simulink model "APP_MyApplication"  (R2018b)
settings: Solver=VariableStepDiscrete  StartTime=0.0  StopTime=10  RelTol=1e-3
PreLoadFcn:
  | if(exist('MBDS_ModelCallback', 'file')), MBDS_ModelCallback('PreLoad'); end;
PostLoadFcn:
  | if(exist('MBDS_ModelCallback', 'file')), MBDS_ModelCallback('PostLoad'); end;
InitFcn:
  | if(exist('MBDS_ModelCallback', 'file')), MBDS_ModelCallback('Init'); end;
StartFcn:
  | if(exist('MBDS_ModelCallback', 'file')), MBDS_ModelCallback('Start'); end;
StopFcn:
  | if(exist('MBDS_ModelCallback', 'file')), MBDS_ModelCallback('Stop'); end;
undefined symbols (not defined in the file): sigbuilder_block, Ts
libraries: KIBES_Signal x499, simulink x8
(part 4 of 10)

== system APP_MyApplication/Model/APP_MyApplication_/DTC List ==
  note: array
  Constant1 : Constant  InitFcn=|  Value=10  OutDataTypeStr=uint8
      | if(exist('MBDS_BlockCallback', 'file'))
      |    MBDS_BlockCallback('Update', gcb);  
      | end
  Constant7 : Constant  InitFcn=|  OutDataTypeStr=uint8
      | if(exist('MBDS_BlockCallback', 'file'))
      |    MBDS_BlockCallback('Update', gcb);  
      | end
  OR1 : Subsystem  InitFcn=|  mask(OR){MBDS_LibraryBlock=on, BitwiseMode=off, Inputs=2, UseBitMask=off, BitMask='A1', OutDataTypeStr=Inherit: Inherit via back propagation, MBDS_BlockVersion=07.21.05}
      | if(exist('MBDS_BlockCallback', 'file'))
      |    MBDS_BlockCallback('Update', gcb);
      | end
      mask prompts: MBDS_LibraryBlock "MBDS library block"; BitwiseMode "Use 'bitwise' mode"; Inputs "Number of input ports:"; UseBitMask "Use bit mask"; BitMask "Bit mask:"; OutDataTypeStr "Output data type:"; MBDS_BlockVersion "Version:"
      mask help: Logical or bitwise OR operator. For multiple inputs, operators are applied across the inputs. For a single input, operators are applied across the input vector. In bitwise mode a bit mask can be applied onto single input signals.
      mask init: same as APP_MyApplication/Model/APP_MyApplication_/OR
      mask Help: eval(['open([workdir(''library_dir:''),''\Blockset\help\'',get_param(gcb,''MaskType''),''.html''])'])
      mask Callback BitwiseMode:
      | if(exist('MBDS_BlockCallback', 'file'))
      |    MBDS_BlockCallback('BitwiseMode', gcb);
      | end
      mask Callback Inputs:
      | if(exist('MBDS_BlockCallback', 'file'))
      |    MBDS_BlockCallback('Inputs', gcb);
      | end
      mask Callback UseBitMask:
      | if(exist('MBDS_BlockCallback', 'file'))
      |    MBDS_BlockCallback('UseBitMask', gcb);
      | end
      mask Callback BitMask:
      | if(exist('MBDS_BlockCallback', 'file'))
      |    MBDS_BlockCallback('BitMask', gcb);
      | end
      mask TypeOptions OutDataTypeStr: Inherit: Inherit via back propagation | int8 | uint8 | int16 | uint16 | int32 | uint32 | boolean
      mask Callback OutDataTypeStr:
      | % Adopt Value
      | if(exist('MBDS_BlockCallback', 'file'))
      |    MBDS_BlockCallback('OutDataTypeStr', gcb);
      | end
      mask DialogControl ParameterTabVar0 Prompt: Main
      mask DialogControl ParameterTabVar01 Prompt: Signal Attributes
      mask DialogControl ParameterTabVar012 Prompt: Version
      mask Display:
      | % Show icon or block text
      | if(UseBitMask)
      |    if(isnumeric(BitMask))
      |       BitMaskString = ['0x',dec2hex(floor(BitMask))];
      |    elseif(ischar(BitMask))
      |       BitMaskString = ['0x',upper(BitMask)];
      |    else
      |       BitMaskString = '???';
      |    end
      |    disp(sprintf(['OR\n', BitMaskString]))
      | else
      |    disp('OR')
      | end
  in_DtcList.DTCList.DTClistType : KIBES_Signal/KIBES_Signal  MBDS_LibraryBlock=on  DatabaseKey=268  SignalName=DtcList.DTCList.DTClistType  SymbolName=DtcList_DTCList_DTClistType_000268  DataType=uint8  Init=[0 0 0 0 0 0 0 0 0 0]  Slope=1  Bias=0  DataSize=10  fpDataType=uint8  BlockIOType=Inport  DeviceType=0
  in_DtcList.DTCList.f_DTClistECUaddress : KIBES_Signal/KIBES_Signal  MBDS_LibraryBlock=on  DatabaseKey=241  SignalName=DtcList.DTCList.f_DTClistECUaddress  SymbolName=DtcList_DTCList_f_DTClistECUaddress_000241  DataType=uint8  Init=[0 0 0 0 0 0 0 0 0 0]  Slope=1  Bias=0  DataSize=10  fpDataType=uint8  BlockIOType=Inport  DeviceType=0
  in_DtcList.DTCList.f_DTClistFMI : KIBES_Signal/KIBES_Signal  MBDS_LibraryBlock=on  DatabaseKey=245  SignalName=DtcList.DTCList.f_DTClistFMI  SymbolName=DtcList_DTCList_f_DTClistFMI_000245  DataType=uint8  Init=[0 0 0 0 0 0 0 0 0 0]  Slope=1  Bias=0  DataSize=10  fpDataType=uint8  BlockIOType=Inport  DeviceType=0
  in_DtcList.DTCList.f_DTClistFirstEntry : KIBES_Signal/KIBES_Signal  MBDS_LibraryBlock=on  DatabaseKey=244  SignalName=DtcList.DTCList.f_DTClistFirstEntry  SymbolName=DtcList_DTCList_f_DTClistFirstEntry_000244  DataType=boolean  Init=0  Slope=1  Bias=0  DataSize=1  fpDataType=boolean  BlockIOType=Inport  DeviceType=0
  in_DtcList.DTCList.f_DTClistLastEntry : KIBES_Signal/KIBES_Signal  MBDS_LibraryBlock=on  DatabaseKey=246  SignalName=DtcList.DTCList.f_DTClistLastEntry  SymbolName=DtcList_DTCList_f_DTClistLastEntry_000246  DataType=boolean  Init=0  Slope=1  Bias=0  DataSize=1  fpDataType=boolean  BlockIOType=Inport  DeviceType=0
  in_DtcList.DTCList.f_DTClistNumOfEntries : KIBES_Signal/KIBES_Signal  MBDS_LibraryBlock=on  DatabaseKey=248  SignalName=DtcList.DTCList.f_DTClistNumOfEntries  SymbolName=DtcList_DTCList_f_DTClistNumOfEntries_000248  DataType=uint16  Init=0  Slope=1  Bias=0  DataSize=1  fpDataType=uint16  BlockIOType=Inport  DeviceType=0
  in_DtcList.DTCList.f_DTClistOCC : KIBES_Signal/KIBES_Signal  MBDS_LibraryBlock=on  DatabaseKey=249  SignalName=DtcList.DTCList.f_DTClistOCC  SymbolName=DtcList_DTCList_f_DTClistOCC_000249  DataType=uint8  Init=[0 0 0 0 0 0 0 0 0 0]  Slope=1  Bias=0  DataSize=10  fpDataType=uint8  BlockIOType=Inport  DeviceType=0
  in_DtcList.DTCList.f_DTClistPrio : KIBES_Signal/KIBES_Signal  MBDS_LibraryBlock=on  DatabaseKey=251  SignalName=DtcList.DTCList.f_DTClistPrio  SymbolName=DtcList_DTCList_f_DTClistPrio_000251  DataType=uint8  Init=[0 0 0 0 0 0 0 0 0 0]  Slope=1  Bias=0  DataSize=10  fpDataType=uint8  BlockIOType=Inport  DeviceType=0
  in_DtcList.DTCList.f_DTClistSPN : KIBES_Signal/KIBES_Signal  MBDS_LibraryBlock=on  DatabaseKey=252  SignalName=DtcList.DTCList.f_DTClistSPN  SymbolName=DtcList_DTCList_f_DTClistSPN_000252  DataType=uint32  Init=[0 0 0 0 0 0 0 0 0 0]  Slope=1  Bias=0  DataSize=10  fpDataType=uint32  BlockIOType=Inport  DeviceType=0
  in_IN_DIG_02_DriverDoor : KIBES_Signal/KIBES_Signal  MBDS_LibraryBlock=on  DatabaseKey=215  SignalName=IN_DIG_02_DriverDoor  SymbolName=IN_DIG_02_DriverDoor_000215  DataType=boolean  Init=0  Slope=1  Bias=0  DataSize=1  fpDataType=boolean  BlockIOType=Inport  DeviceType=0
  in_STIMD.ListDtcEcuAddrMask : KIBES_Signal/KIBES_Signal  MBDS_LibraryBlock=on  DatabaseKey=254  SignalName=STIMD.ListDtcEcuAddrMask  SymbolName=STIMD_ListDtcEcuAddrMask_000254  DataType=uint8  Init=255  Slope=1  Bias=0  DataSize=1  fpDataType=uint8  BlockIOType=Inport  DeviceType=2
  in_STIMD.ListDtcEnable : KIBES_Signal/KIBES_Signal  MBDS_LibraryBlock=on  DatabaseKey=255  SignalName=STIMD.ListDtcEnable  SymbolName=STIMD_ListDtcEnable_000255  DataType=boolean  Init=0  Slope=1  Bias=0  DataSize=1  fpDataType=boolean  BlockIOType=Inport  DeviceType=2
  in_STIMD.ListDtcNextEntry : KIBES_Signal/KIBES_Signal  MBDS_LibraryBlock=on  DatabaseKey=256  SignalName=STIMD.ListDtcNextEntry  SymbolName=STIMD_ListDtcNextEntry_000256  DataType=boolean  Init=0  Slope=1  Bias=0  DataSize=1  fpDataType=boolean  BlockIOType=Inport  DeviceType=2
  in_STIMD.ListDtcPrevEntry : KIBES_Signal/KIBES_Signal  MBDS_LibraryBlock=on  DatabaseKey=257  SignalName=STIMD.ListDtcPrevEntry  SymbolName=STIMD_ListDtcPrevEntry_000257  DataType=boolean  Init=0  Slope=1  Bias=0  DataSize=1  fpDataType=boolean  BlockIOType=Inport  DeviceType=2
  in_STIMD.ListDtcSelectCanChannel : KIBES_Signal/KIBES_Signal  MBDS_LibraryBlock=on  DatabaseKey=450  SignalName=STIMD.ListDtcSelectCanChannel  SymbolName=STIMD_ListDtcSelectCanChannel_000450  DataType=uint8  Init=10  Slope=1  Bias=0  DataSize=1  fpDataType=uint8  BlockIOType=Inport  DeviceType=2
  in_STIMD.ListDtcStatusMask : KIBES_Signal/KIBES_Signal  MBDS_LibraryBlock=on  DatabaseKey=258  SignalName=STIMD.ListDtcStatusMask  SymbolName=STIMD_ListDtcStatusMask_000258  DataType=uint8  Init=1  Slope=1  Bias=0  DataSize=1  fpDataType=uint8  BlockIOType=Inport  DeviceType=2
  out_DtcList.DTCList.SelectCANChannel : KIBES_Signal/KIBES_Signal  MBDS_LibraryBlock=on  DatabaseKey=269  SignalName=DtcList.DTCList.SelectCANChannel  SymbolName=DtcList_DTCList_SelectCANChannel_000269  DataType=uint8  Init=0  Slope=1  Bias=0  DataSize=1  fpDataType=uint8  BlockIOType=Outport  DeviceType=0
  out_DtcList.DTCList.f_DTClistECUaddrMask : KIBES_Signal/KIBES_Signal  MBDS_LibraryBlock=on  DatabaseKey=242  SignalName=DtcList.DTCList.f_DTClistECUaddrMask  SymbolName=DtcList_DTCList_f_DTClistECUaddrMask_000242  DataType=uint8  Init=0  Slope=1  Bias=0  DataSize=1  fpDataType=uint8  BlockIOType=Outport  DeviceType=0
  out_DtcList.DTCList.f_DTClistEna : KIBES_Signal/KIBES_Signal  MBDS_LibraryBlock=on  DatabaseKey=243  SignalName=DtcList.DTCList.f_DTClistEna  SymbolName=DtcList_DTCList_f_DTClistEna_000243  DataType=boolean  Init=0  Slope=1  Bias=0  DataSize=1  fpDataType=boolean  BlockIOType=Outport  DeviceType=0
  out_DtcList.DTCList.f_DTClistNextEntry : KIBES_Signal/KIBES_Signal  MBDS_LibraryBlock=on  DatabaseKey=247  SignalName=DtcList.DTCList.f_DTClistNextEntry  SymbolName=DtcList_DTCList_f_DTClistNextEntry_000247  DataType=boolean  Init=0  Slope=1  Bias=0  DataSize=1  fpDataType=boolean  BlockIOType=Outport  DeviceType=0
  out_DtcList.DTCList.f_DTClistPrevEntry : KIBES_Signal/KIBES_Signal  MBDS_LibraryBlock=on  DatabaseKey=250  SignalName=DtcList.DTCList.f_DTClistPrevEntry  SymbolName=DtcList_DTCList_f_DTClistPrevEntry_000250  DataType=boolean  Init=0  Slope=1  Bias=0  DataSize=1  fpDataType=boolean  BlockIOType=Outport  DeviceType=0
  out_DtcList.DTCList.f_DTClistStatusMask : KIBES_Signal/KIBES_Signal  MBDS_LibraryBlock=on  DatabaseKey=253  SignalName=DtcList.DTCList.f_DTClistStatusMask  SymbolName=DtcList_DTCList_f_DTClistStatusMask_000253  DataType=uint8  Init=0  Slope=1  Bias=0  DataSize=1  fpDataType=uint8  BlockIOType=Outport  DeviceType=0
  wires:
  in_STIMD.ListDtcEcuAddrMask/1 -> out_DtcList.DTCList.f_DTClistECUaddrMask/1
  in_STIMD.ListDtcNextEntry/1 -> out_DtcList.DTCList.f_DTClistNextEntry/1
  in_STIMD.ListDtcPrevEntry/1 -> out_DtcList.DTCList.f_DTClistPrevEntry/1
  OR1/1(y) -> out_DtcList.DTCList.f_DTClistEna/1
  in_STIMD.ListDtcEnable/1 -> OR1/1(u1)
  in_IN_DIG_02_DriverDoor/1 -> OR1/2(u2)
  in_STIMD.ListDtcStatusMask/1 -> out_DtcList.DTCList.f_DTClistStatusMask/1
  in_STIMD.ListDtcSelectCanChannel/1 -> out_DtcList.DTCList.SelectCANChannel/1

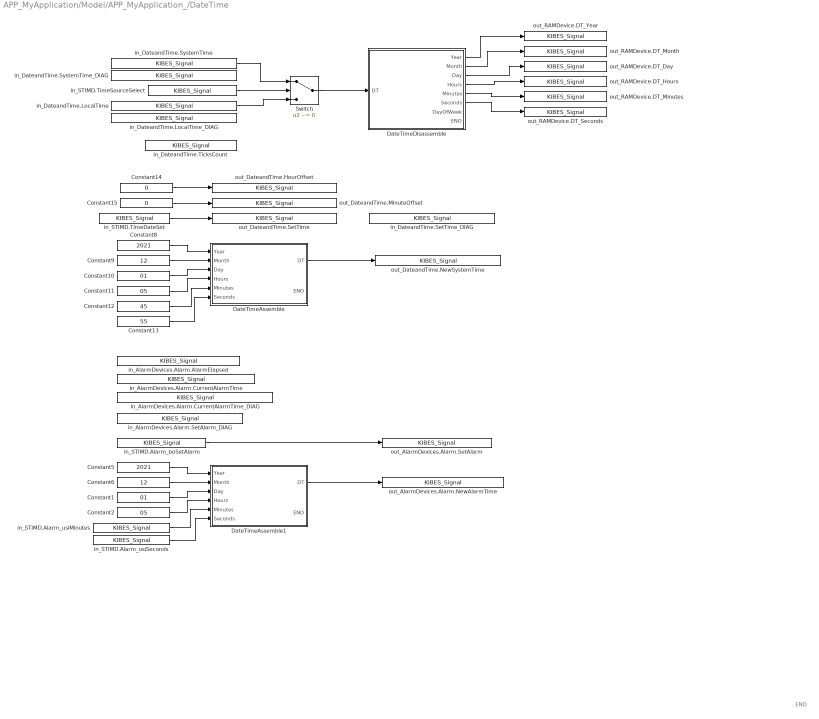
== system APP_MyApplication/Model/APP_MyApplication_/DateTime ==
  note: END
  Constant1 : Constant  InitFcn=|  Value=01  OutDataTypeStr=uint8
      | if(exist('MBDS_BlockCallback', 'file'))
      |    MBDS_BlockCallback('Update', gcb);  
      | end
  Constant10 : Constant  InitFcn=|  Value=01  OutDataTypeStr=uint8
      | if(exist('MBDS_BlockCallback', 'file'))
      |    MBDS_BlockCallback('Update', gcb);  
      | end
  Constant11 : Constant  InitFcn=|  Value=05  OutDataTypeStr=uint8
      | if(exist('MBDS_BlockCallback', 'file'))
      |    MBDS_BlockCallback('Update', gcb);  
      | end
  Constant12 : Constant  InitFcn=|  Value=45  OutDataTypeStr=uint8
      | if(exist('MBDS_BlockCallback', 'file'))
      |    MBDS_BlockCallback('Update', gcb);  
      | end
  Constant13 : Constant  InitFcn=|  Value=55  OutDataTypeStr=uint8
      | if(exist('MBDS_BlockCallback', 'file'))
      |    MBDS_BlockCallback('Update', gcb);  
      | end
  Constant14 : Constant  InitFcn=|  Value=0  OutDataTypeStr=int8
      | if(exist('MBDS_BlockCallback', 'file'))
      |    MBDS_BlockCallback('Update', gcb);  
      | end
  Constant15 : Constant  InitFcn=|  Value=0  OutDataTypeStr=int8
      | if(exist('MBDS_BlockCallback', 'file'))
      |    MBDS_BlockCallback('Update', gcb);  
      | end
  Constant2 : Constant  InitFcn=|  Value=05  OutDataTypeStr=uint8
      | if(exist('MBDS_BlockCallback', 'file'))
      |    MBDS_BlockCallback('Update', gcb);  
      | end
  Constant5 : Constant  InitFcn=|  Value=2021  OutDataTypeStr=uint16
      | if(exist('MBDS_BlockCallback', 'file'))
      |    MBDS_BlockCallback('Update', gcb);  
      | end
  Constant6 : Constant  InitFcn=|  Value=12  OutDataTypeStr=uint8
      | if(exist('MBDS_BlockCallback', 'file'))
      |    MBDS_BlockCallback('Update', gcb);  
      | end
  Constant8 : Constant  InitFcn=|  Value=2021  OutDataTypeStr=uint16
      | if(exist('MBDS_BlockCallback', 'file'))
      |    MBDS_BlockCallback('Update', gcb);  
      | end
  Constant9 : Constant  InitFcn=|  Value=12  OutDataTypeStr=uint8
      | if(exist('MBDS_BlockCallback', 'file'))
      |    MBDS_BlockCallback('Update', gcb);  
      | end
  DateTimeAssemble : Subsystem  mask(DateTimeAssemble){MBDS_LibraryBlock=on, ENO_Enabled=on, MBDS_BlockVersion=07.21.06}
      mask prompts: MBDS_LibraryBlock "MBDS library block"; ENO_Enabled "Show ENO port"; MBDS_BlockVersion "Block version:"
      mask help: Assembles a date_time signal from individual date and time components. The input values are restricted to their ranges (refer to the block help). If an input is out of range the ENO output is set to false.
      mask init: same as APP_MyApplication/Model/APP_MyApplication_/OR
      mask Help: eval(['open([workdir(''Library_Dir:''),''\Blockset\Help\'',get_param(gcb,''MaskType''),''.html''])']);
      mask DialogControl Container4 Prompt: Main
      mask DialogControl Container5 Prompt: Version
      mask Display:
      | % Show block text
      | disp(sprintf('DateTime\nAssemble'));
      | 
      | % Display port labels
      | port_label('input', 1, 'Year');
      | port_label('input', 2, 'Month');
      | port_label('input', 3, 'Day');
      | port_label('input', 4, 'Hours');
      | port_label('input', 5, 'Minutes');
      | port_label('input', 6, 'Seconds');
      | port_label('output', 1, 'DT');
      | port_label('output', 2, 'ENO');
  DateTimeAssemble1 : Subsystem  mask(DateTimeAssemble){MBDS_LibraryBlock=on, ENO_Enabled=on, MBDS_BlockVersion=07.21.06}
      mask prompts: MBDS_LibraryBlock "MBDS library block"; ENO_Enabled "Show ENO port"; MBDS_BlockVersion "Block version:"
      mask help: Assembles a date_time signal from individual date and time components. The input values are restricted to their ranges (refer to the block help). If an input is out of range the ENO output is set to false.
      mask init: same as APP_MyApplication/Model/APP_MyApplication_/OR
      mask Help: eval(['open([workdir(''Library_Dir:''),''\Blockset\Help\'',get_param(gcb,''MaskType''),''.html''])']);
      mask DialogControl Container4 Prompt: Main
      mask DialogControl Container5 Prompt: Version
      mask Display:
      | % Show block text
      | disp(sprintf('DateTime\nAssemble'));
      | 
      | % Display port labels
      | port_label('input', 1, 'Year');
      | port_label('input', 2, 'Month');
      | port_label('input', 3, 'Day');
      | port_label('input', 4, 'Hours');
      | port_label('input', 5, 'Minutes');
      | port_label('input', 6, 'Seconds');
      | port_label('output', 1, 'DT');
      | port_label('output', 2, 'ENO');
  DateTimeDisassemble : Subsystem  mask(DateTimeDisassemble){MBDS_LibraryBlock=on, ENO_Enabled=on, MBDS_BlockVersion=07.21.06}
      mask prompts: MBDS_LibraryBlock "MBDS library block"; ENO_Enabled "Show ENO port"; MBDS_BlockVersion "Block version:"
      mask help: Disassembles a date_time signal into its date time components, i.e. year, month, day, hour, minute, second. Additionally the day of week number is output. If the input signal is invalid the ENO output is false.
      mask init: same as APP_MyApplication/Model/APP_MyApplication_/OR
      mask Help: eval(['open([workdir(''Library_Dir:''),''\Blockset\Help\'',get_param(gcb,''MaskType''),''.html''])']);
      mask DialogControl Container8 Prompt: Main
      mask DialogControl Container11 Prompt: Version
      mask Display:
      | % Show block text
      | disp(sprintf('DateTime\nDisassemble'));
      | 
      | % Display port labels
      | port_label('input', 1, 'DT');
      | port_label('output', 1, 'Year');
      | port_label('output', 2, 'Month');
      | port_label('output', 3, 'Day');
      | port_label('output', 4, 'Hours');
      | port_label('output', 5, 'Minutes');
      | port_label('output', 6, 'Seconds');
      | port_label('output', 7, 'DayOfWeek');
      | port_label('output', 8, 'ENO');
  Switch : Switch  InitFcn=|  Criteria=u2 ~= 0  OutDataTypeStr=Inherit: Inherit via back propagation  mask(Switch){MBDS_LibraryBlock=on, OutDataTypeStr_=Inherit: Inherit via back propagation, SaturateOnIntegerOverflow_=off, InputSameDT_=off, MBDS_BlockVersion=07.21.05}
      | if(exist('MBDS_BlockCallback', 'file'))
      |    MBDS_BlockCallback('Update', gcb);  
      | end
      mask prompts: MBDS_LibraryBlock "MBDS library block"; OutDataTypeStr_ "Output data type:"; SaturateOnIntegerOverflow_ "Saturate on integer overflow"; InputSameDT_ "Require all inputs to have the same data type"; MBDS_BlockVersion "Block version:"
      mask help: Pass through input 1 when input 2 is not equal to zero; otherwise pass through input 3. The inputs are numbered top to bottom (or left to right). The first and third input ports are data ports, and the second input port is the control port.
      mask init: same as APP_MyApplication/Model/APP_MyApplication_/OR
      mask Help: eval(['open([workdir(''library_dir:''),''\Blockset\help\'',get_param(gcb,''MaskType''),''.html''])'])
      mask TypeOptions OutDataTypeStr_: Inherit: Inherit via back propagation | single | int8 | uint8 | int16 | uint16 | int32 | uint32
      mask DialogControl ParameterTabVar0 Prompt: Signal Attributes
      mask DialogControl ParameterTabVar01 Prompt: Version
  in_AlarmDevices.Alarm.AlarmElapsed : KIBES_Signal/KIBES_Signal  MBDS_LibraryBlock=on  DatabaseKey=621  SignalName=AlarmDevices.Alarm.AlarmElapsed  SymbolName=AlarmDevices_Alarm_AlarmElapsed_000621  DataType=boolean  Init=0  Slope=1  Bias=0  DataSize=1  fpDataType=boolean  BlockIOType=Inport  DeviceType=0
  in_AlarmDevices.Alarm.CurrentAlarmTime : KIBES_Signal/KIBES_Signal  MBDS_LibraryBlock=on  DatabaseKey=623  SignalName=AlarmDevices.Alarm.CurrentAlarmTime  SymbolName=AlarmDevices_Alarm_CurrentAlarmTime_000623  DataType=uint32  Init=0  Slope=1  Bias=0  DataSize=1  fpDataType=uint32  BlockIOType=Inport  DeviceType=0
  in_AlarmDevices.Alarm.CurrentAlarmTime_DIAG : KIBES_Signal/KIBES_Signal  MBDS_LibraryBlock=on  DatabaseKey=624  SignalName=AlarmDevices.Alarm.CurrentAlarmTime_DIAG  SymbolName=AlarmDevices_Alarm_CurrentAlarmTime_DIAG_000624  DataType=uint16  Init=1  Slope=1  Bias=0  DataSize=1  fpDataType=uint16  BlockIOType=Inport  DeviceType=0
  in_AlarmDevices.Alarm.SetAlarm_DIAG : KIBES_Signal/KIBES_Signal  MBDS_LibraryBlock=on  DatabaseKey=634  SignalName=AlarmDevices.Alarm.SetAlarm_DIAG  SymbolName=AlarmDevices_Alarm_SetAlarm_DIAG_000634  DataType=uint16  Init=1  Slope=1  Bias=0  DataSize=1  fpDataType=uint16  BlockIOType=Inport  DeviceType=0
  in_DateandTime.LocalTime : KIBES_Signal/KIBES_Signal  MBDS_LibraryBlock=on  DatabaseKey=415  SignalName=DateandTime.LocalTime  SymbolName=DateandTime_LocalTime_000415  DataType=uint32  Init=0  Slope=1  Bias=0  DataSize=1  fpDataType=uint32  BlockIOType=Inport  DeviceType=0
  in_DateandTime.LocalTime_DIAG : KIBES_Signal/KIBES_Signal  MBDS_LibraryBlock=on  DatabaseKey=418  SignalName=DateandTime.LocalTime_DIAG  SymbolName=DateandTime_LocalTime_DIAG_000418  DataType=uint16  Init=1  Slope=1  Bias=0  DataSize=1  fpDataType=uint16  BlockIOType=Inport  DeviceType=0
  in_DateandTime.SetTime_DIAG : KIBES_Signal/KIBES_Signal  MBDS_LibraryBlock=on  DatabaseKey=410  SignalName=DateandTime.SetTime_DIAG  SymbolName=DateandTime_SetTime_DIAG_000410  DataType=uint16  Init=1  Slope=1  Bias=0  DataSize=1  fpDataType=uint16  BlockIOType=Inport  DeviceType=0
  in_DateandTime.SystemTime : KIBES_Signal/KIBES_Signal  MBDS_LibraryBlock=on  DatabaseKey=412  SignalName=DateandTime.SystemTime  SymbolName=DateandTime_SystemTime_000412  DataType=uint32  Init=0  Slope=1  Bias=0  DataSize=1  fpDataType=uint32  BlockIOType=Inport  DeviceType=0
  in_DateandTime.SystemTime_DIAG : KIBES_Signal/KIBES_Signal  MBDS_LibraryBlock=on  DatabaseKey=413  SignalName=DateandTime.SystemTime_DIAG  SymbolName=DateandTime_SystemTime_DIAG_000413  DataType=uint16  Init=1  Slope=1  Bias=0  DataSize=1  fpDataType=uint16  BlockIOType=Inport  DeviceType=0
  in_DateandTime.TicksCount : KIBES_Signal/KIBES_Signal  MBDS_LibraryBlock=on  DatabaseKey=414  SignalName=DateandTime.TicksCount  SymbolName=DateandTime_TicksCount_000414  DataType=uint32  Init=0  Slope=1  Bias=0  DataSize=1  fpDataType=uint32  BlockIOType=Inport  DeviceType=0
  in_STIMD.Alarm_boSetAlarm : KIBES_Signal/KIBES_Signal  MBDS_LibraryBlock=on  DatabaseKey=627  SignalName=STIMD.Alarm_boSetAlarm  SymbolName=STIMD_Alarm_boSetAlarm_000627  DataType=boolean  Init=0  Slope=1  Bias=0  DataSize=1  fpDataType=boolean  BlockIOType=Inport  DeviceType=2
  in_STIMD.Alarm_usiMinutes : KIBES_Signal/KIBES_Signal  MBDS_LibraryBlock=on  DatabaseKey=628  SignalName=STIMD.Alarm_usiMinutes  SymbolName=STIMD_Alarm_usiMinutes_000628  DataType=uint8  Init=0  Slope=1  Bias=0  DataSize=1  fpDataType=uint8  BlockIOType=Inport  DeviceType=2
  in_STIMD.Alarm_usiSeconds : KIBES_Signal/KIBES_Signal  MBDS_LibraryBlock=on  DatabaseKey=630  SignalName=STIMD.Alarm_usiSeconds  SymbolName=STIMD_Alarm_usiSeconds_000630  DataType=uint8  Init=0  Slope=1  Bias=0  DataSize=1  fpDataType=uint8  BlockIOType=Inport  DeviceType=2
  in_STIMD.TimeDateSet : KIBES_Signal/KIBES_Signal  MBDS_LibraryBlock=on  DatabaseKey=420  SignalName=STIMD.TimeDateSet  SymbolName=STIMD_TimeDateSet_000420  DataType=boolean  Init=0  Slope=1  Bias=0  DataSize=1  fpDataType=boolean  BlockIOType=Inport  DeviceType=2
  in_STIMD.TimeSourceSelect : KIBES_Signal/KIBES_Signal  MBDS_LibraryBlock=on  DatabaseKey=620  SignalName=STIMD.TimeSourceSelect  SymbolName=STIMD_TimeSourceSelect_000620  DataType=boolean  Init=0  Slope=1  Bias=0  DataSize=1  fpDataType=boolean  BlockIOType=Inport  DeviceType=2
  out_AlarmDevices.Alarm.NewAlarmTime : KIBES_Signal/KIBES_Signal  MBDS_LibraryBlock=on  DatabaseKey=625  SignalName=AlarmDevices.Alarm.NewAlarmTime  SymbolName=AlarmDevices_Alarm_NewAlarmTime_000625  DataType=uint32  Init=0  Slope=1  Bias=0  DataSize=1  fpDataType=uint32  BlockIOType=Outport  DeviceType=0
  out_AlarmDevices.Alarm.SetAlarm : KIBES_Signal/KIBES_Signal  MBDS_LibraryBlock=on  DatabaseKey=626  SignalName=AlarmDevices.Alarm.SetAlarm  SymbolName=AlarmDevices_Alarm_SetAlarm_000626  DataType=boolean  Init=0  Slope=1  Bias=0  DataSize=1  fpDataType=boolean  BlockIOType=Outport  DeviceType=0
  out_DateandTime.HourOffset : KIBES_Signal/KIBES_Signal  MBDS_LibraryBlock=on  DatabaseKey=416  SignalName=DateandTime.HourOffset  SymbolName=DateandTime_HourOffset_000416  DataType=int8  Init=0  Slope=1  Bias=0  DataSize=1  fpDataType=int8  BlockIOType=Outport  DeviceType=0
  out_DateandTime.MinuteOffset : KIBES_Signal/KIBES_Signal  MBDS_LibraryBlock=on  DatabaseKey=419  SignalName=DateandTime.MinuteOffset  SymbolName=DateandTime_MinuteOffset_000419  DataType=int8  Init=0  Slope=1  Bias=0  DataSize=1  fpDataType=int8  BlockIOType=Outport  DeviceType=0
  out_DateandTime.NewSystemTime : KIBES_Signal/KIBES_Signal  MBDS_LibraryBlock=on  DatabaseKey=417  SignalName=DateandTime.NewSystemTime  SymbolName=DateandTime_NewSystemTime_000417  DataType=uint32  Init=0  Slope=1  Bias=0  DataSize=1  fpDataType=uint32  BlockIOType=Outport  DeviceType=0
  out_DateandTime.SetTime : KIBES_Signal/KIBES_Signal  MBDS_LibraryBlock=on  DatabaseKey=411  SignalName=DateandTime.SetTime  SymbolName=DateandTime_SetTime_000411  DataType=boolean  Init=0  Slope=1  Bias=0  DataSize=1  fpDataType=boolean  BlockIOType=Outport  DeviceType=0
  out_RAMDevice.DT_Day : KIBES_Signal/KIBES_Signal  MBDS_LibraryBlock=on  DatabaseKey=424  SignalName=RAMDevice.DT_Day  SymbolName=RAMDevice_DT_Day_000424  DataType=uint8  Init=0  Slope=1  Bias=0  DataSize=1  fpDataType=uint8  BlockIOType=Outport  DeviceType=0
  out_RAMDevice.DT_Hours : KIBES_Signal/KIBES_Signal  MBDS_LibraryBlock=on  DatabaseKey=423  SignalName=RAMDevice.DT_Hours  SymbolName=RAMDevice_DT_Hours_000423  DataType=uint8  Init=0  Slope=1  Bias=0  DataSize=1  fpDataType=uint8  BlockIOType=Outport  DeviceType=0
  out_RAMDevice.DT_Minutes : KIBES_Signal/KIBES_Signal  MBDS_LibraryBlock=on  DatabaseKey=425  SignalName=RAMDevice.DT_Minutes  SymbolName=RAMDevice_DT_Minutes_000425  DataType=uint8  Init=0  Slope=1  Bias=0  DataSize=1  fpDataType=uint8  BlockIOType=Outport  DeviceType=0
  out_RAMDevice.DT_Month : KIBES_Signal/KIBES_Signal  MBDS_LibraryBlock=on  DatabaseKey=422  SignalName=RAMDevice.DT_Month  SymbolName=RAMDevice_DT_Month_000422  DataType=uint8  Init=0  Slope=1  Bias=0  DataSize=1  fpDataType=uint8  BlockIOType=Outport  DeviceType=0
  out_RAMDevice.DT_Seconds : KIBES_Signal/KIBES_Signal  MBDS_LibraryBlock=on  DatabaseKey=426  SignalName=RAMDevice.DT_Seconds  SymbolName=RAMDevice_DT_Seconds_000426  DataType=uint8  Init=0  Slope=1  Bias=0  DataSize=1  fpDataType=uint8  BlockIOType=Outport  DeviceType=0
  out_RAMDevice.DT_Year : KIBES_Signal/KIBES_Signal  MBDS_LibraryBlock=on  DatabaseKey=421  SignalName=RAMDevice.DT_Year  SymbolName=RAMDevice_DT_Year_000421  DataType=uint16  Init=0  Slope=1  Bias=0  DataSize=1  fpDataType=uint16  BlockIOType=Outport  DeviceType=0
  wires:
  DateTimeAssemble/1(DT) -> out_DateandTime.NewSystemTime/1
  Constant8/1 -> DateTimeAssemble/1(Year)
  Constant9/1 -> DateTimeAssemble/2(Month)
  Constant10/1 -> DateTimeAssemble/3(Day)
  Constant11/1 -> DateTimeAssemble/4(Hours)
  Constant12/1 -> DateTimeAssemble/5(Minutes)
  Constant13/1 -> DateTimeAssemble/6(Seconds)
  Constant14/1 -> out_DateandTime.HourOffset/1
  Constant15/1 -> out_DateandTime.MinuteOffset/1
  in_STIMD.TimeDateSet/1 -> out_DateandTime.SetTime/1
  DateTimeDisassemble/2(Month) -> out_RAMDevice.DT_Month/1
  DateTimeDisassemble/1(Year) -> out_RAMDevice.DT_Year/1
  DateTimeDisassemble/5(Minutes) -> out_RAMDevice.DT_Minutes/1
  DateTimeDisassemble/4(Hours) -> out_RAMDevice.DT_Hours/1
  DateTimeDisassemble/3(Day) -> out_RAMDevice.DT_Day/1
  DateTimeDisassemble/6(Seconds) -> out_RAMDevice.DT_Seconds/1
  in_DateandTime.SystemTime/1 -> Switch/1
  in_DateandTime.LocalTime/1 -> Switch/3
  Switch/1 -> DateTimeDisassemble/1(DT)
  in_STIMD.TimeSourceSelect/1 -> Switch/2
  Constant2/1 -> DateTimeAssemble1/4(Hours)
  Constant1/1 -> DateTimeAssemble1/3(Day)
  Constant6/1 -> DateTimeAssemble1/2(Month)
  Constant5/1 -> DateTimeAssemble1/1(Year)
  DateTimeAssemble1/1(DT) -> out_AlarmDevices.Alarm.NewAlarmTime/1
  in_STIMD.Alarm_boSetAlarm/1 -> out_AlarmDevices.Alarm.SetAlarm/1
  in_STIMD.Alarm_usiMinutes/1 -> DateTimeAssemble1/5(Minutes)
  in_STIMD.Alarm_usiSeconds/1 -> DateTimeAssemble1/6(Seconds)

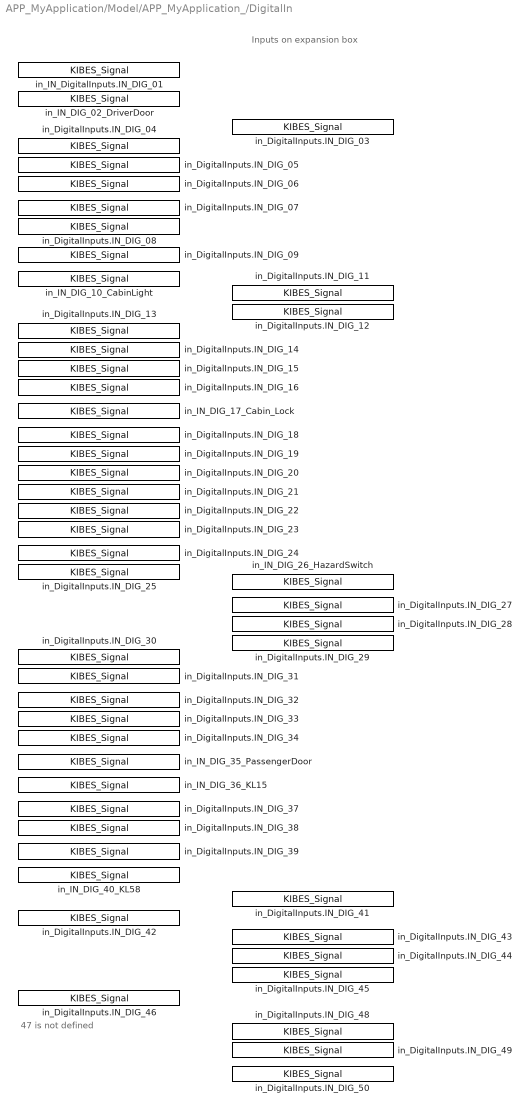
== system APP_MyApplication/Model/APP_MyApplication_/DigitalIn ==
  note: 47 is not defined
  note: Inputs on expansion box
  in_DigitalInputs.IN_DIG_03 : KIBES_Signal/KIBES_Signal  MBDS_LibraryBlock=on  DatabaseKey=456  SignalName=DigitalInputs.IN_DIG_03  SymbolName=DigitalInputs_IN_DIG_03_000456  DataType=boolean  Init=0  Slope=1  Bias=0  DataSize=1  fpDataType=boolean  BlockIOType=Inport  DeviceType=0
  in_DigitalInputs.IN_DIG_04 : KIBES_Signal/KIBES_Signal  MBDS_LibraryBlock=on  DatabaseKey=461  SignalName=DigitalInputs.IN_DIG_04  SymbolName=DigitalInputs_IN_DIG_04_000461  DataType=boolean  Init=0  Slope=1  Bias=0  DataSize=1  fpDataType=boolean  BlockIOType=Inport  DeviceType=0
  in_DigitalInputs.IN_DIG_05 : KIBES_Signal/KIBES_Signal  MBDS_LibraryBlock=on  DatabaseKey=462  SignalName=DigitalInputs.IN_DIG_05  SymbolName=DigitalInputs_IN_DIG_05_000462  DataType=boolean  Init=0  Slope=1  Bias=0  DataSize=1  fpDataType=boolean  BlockIOType=Inport  DeviceType=0
  in_DigitalInputs.IN_DIG_06 : KIBES_Signal/KIBES_Signal  MBDS_LibraryBlock=on  DatabaseKey=463  SignalName=DigitalInputs.IN_DIG_06  SymbolName=DigitalInputs_IN_DIG_06_000463  DataType=boolean  Init=0  Slope=1  Bias=0  DataSize=1  fpDataType=boolean  BlockIOType=Inport  DeviceType=0
  in_DigitalInputs.IN_DIG_07 : KIBES_Signal/KIBES_Signal  MBDS_LibraryBlock=on  DatabaseKey=464  SignalName=DigitalInputs.IN_DIG_07  SymbolName=DigitalInputs_IN_DIG_07_000464  DataType=boolean  Init=0  Slope=1  Bias=0  DataSize=1  fpDataType=boolean  BlockIOType=Inport  DeviceType=0
  in_DigitalInputs.IN_DIG_08 : KIBES_Signal/KIBES_Signal  MBDS_LibraryBlock=on  DatabaseKey=465  SignalName=DigitalInputs.IN_DIG_08  SymbolName=DigitalInputs_IN_DIG_08_000465  DataType=boolean  Init=0  Slope=1  Bias=0  DataSize=1  fpDataType=boolean  BlockIOType=Inport  DeviceType=0
  in_DigitalInputs.IN_DIG_09 : KIBES_Signal/KIBES_Signal  MBDS_LibraryBlock=on  DatabaseKey=457  SignalName=DigitalInputs.IN_DIG_09  SymbolName=DigitalInputs_IN_DIG_09_000457  DataType=boolean  Init=0  Slope=1  Bias=0  DataSize=1  fpDataType=boolean  BlockIOType=Inport  DeviceType=0
  in_DigitalInputs.IN_DIG_11 : KIBES_Signal/KIBES_Signal  MBDS_LibraryBlock=on  DatabaseKey=466  SignalName=DigitalInputs.IN_DIG_11  SymbolName=DigitalInputs_IN_DIG_11_000466  DataType=boolean  Init=0  Slope=1  Bias=0  DataSize=1  fpDataType=boolean  BlockIOType=Inport  DeviceType=0
  in_DigitalInputs.IN_DIG_12 : KIBES_Signal/KIBES_Signal  MBDS_LibraryBlock=on  DatabaseKey=467  SignalName=DigitalInputs.IN_DIG_12  SymbolName=DigitalInputs_IN_DIG_12_000467  DataType=boolean  Init=0  Slope=1  Bias=0  DataSize=1  fpDataType=boolean  BlockIOType=Inport  DeviceType=0
  in_DigitalInputs.IN_DIG_13 : KIBES_Signal/KIBES_Signal  MBDS_LibraryBlock=on  DatabaseKey=468  SignalName=DigitalInputs.IN_DIG_13  SymbolName=DigitalInputs_IN_DIG_13_000468  DataType=boolean  Init=0  Slope=1  Bias=0  DataSize=1  fpDataType=boolean  BlockIOType=Inport  DeviceType=0
  in_DigitalInputs.IN_DIG_14 : KIBES_Signal/KIBES_Signal  MBDS_LibraryBlock=on  DatabaseKey=469  SignalName=DigitalInputs.IN_DIG_14  SymbolName=DigitalInputs_IN_DIG_14_000469  DataType=boolean  Init=0  Slope=1  Bias=0  DataSize=1  fpDataType=boolean  BlockIOType=Inport  DeviceType=0
  in_DigitalInputs.IN_DIG_15 : KIBES_Signal/KIBES_Signal  MBDS_LibraryBlock=on  DatabaseKey=470  SignalName=DigitalInputs.IN_DIG_15  SymbolName=DigitalInputs_IN_DIG_15_000470  DataType=boolean  Init=0  Slope=1  Bias=0  DataSize=1  fpDataType=boolean  BlockIOType=Inport  DeviceType=0
  in_DigitalInputs.IN_DIG_16 : KIBES_Signal/KIBES_Signal  MBDS_LibraryBlock=on  DatabaseKey=471  SignalName=DigitalInputs.IN_DIG_16  SymbolName=DigitalInputs_IN_DIG_16_000471  DataType=boolean  Init=0  Slope=1  Bias=0  DataSize=1  fpDataType=boolean  BlockIOType=Inport  DeviceType=0
  in_DigitalInputs.IN_DIG_18 : KIBES_Signal/KIBES_Signal  MBDS_LibraryBlock=on  DatabaseKey=472  SignalName=DigitalInputs.IN_DIG_18  SymbolName=DigitalInputs_IN_DIG_18_000472  DataType=boolean  Init=0  Slope=1  Bias=0  DataSize=1  fpDataType=boolean  BlockIOType=Inport  DeviceType=0
  in_DigitalInputs.IN_DIG_19 : KIBES_Signal/KIBES_Signal  MBDS_LibraryBlock=on  DatabaseKey=473  SignalName=DigitalInputs.IN_DIG_19  SymbolName=DigitalInputs_IN_DIG_19_000473  DataType=boolean  Init=0  Slope=1  Bias=0  DataSize=1  fpDataType=boolean  BlockIOType=Inport  DeviceType=0
  in_DigitalInputs.IN_DIG_20 : KIBES_Signal/KIBES_Signal  MBDS_LibraryBlock=on  DatabaseKey=474  SignalName=DigitalInputs.IN_DIG_20  SymbolName=DigitalInputs_IN_DIG_20_000474  DataType=boolean  Init=0  Slope=1  Bias=0  DataSize=1  fpDataType=boolean  BlockIOType=Inport  DeviceType=0
  in_DigitalInputs.IN_DIG_21 : KIBES_Signal/KIBES_Signal  MBDS_LibraryBlock=on  DatabaseKey=475  SignalName=DigitalInputs.IN_DIG_21  SymbolName=DigitalInputs_IN_DIG_21_000475  DataType=boolean  Init=0  Slope=1  Bias=0  DataSize=1  fpDataType=boolean  BlockIOType=Inport  DeviceType=0
  in_DigitalInputs.IN_DIG_22 : KIBES_Signal/KIBES_Signal  MBDS_LibraryBlock=on  DatabaseKey=476  SignalName=DigitalInputs.IN_DIG_22  SymbolName=DigitalInputs_IN_DIG_22_000476  DataType=boolean  Init=0  Slope=1  Bias=0  DataSize=1  fpDataType=boolean  BlockIOType=Inport  DeviceType=0
  in_DigitalInputs.IN_DIG_23 : KIBES_Signal/KIBES_Signal  MBDS_LibraryBlock=on  DatabaseKey=477  SignalName=DigitalInputs.IN_DIG_23  SymbolName=DigitalInputs_IN_DIG_23_000477  DataType=boolean  Init=0  Slope=1  Bias=0  DataSize=1  fpDataType=boolean  BlockIOType=Inport  DeviceType=0
  in_DigitalInputs.IN_DIG_24 : KIBES_Signal/KIBES_Signal  MBDS_LibraryBlock=on  DatabaseKey=478  SignalName=DigitalInputs.IN_DIG_24  SymbolName=DigitalInputs_IN_DIG_24_000478  DataType=boolean  Init=0  Slope=1  Bias=0  DataSize=1  fpDataType=boolean  BlockIOType=Inport  DeviceType=0
  in_DigitalInputs.IN_DIG_25 : KIBES_Signal/KIBES_Signal  MBDS_LibraryBlock=on  DatabaseKey=479  SignalName=DigitalInputs.IN_DIG_25  SymbolName=DigitalInputs_IN_DIG_25_000479  DataType=boolean  Init=0  Slope=1  Bias=0  DataSize=1  fpDataType=boolean  BlockIOType=Inport  DeviceType=0
  in_DigitalInputs.IN_DIG_27 : KIBES_Signal/KIBES_Signal  MBDS_LibraryBlock=on  DatabaseKey=458  SignalName=DigitalInputs.IN_DIG_27  SymbolName=DigitalInputs_IN_DIG_27_000458  DataType=boolean  Init=0  Slope=1  Bias=0  DataSize=1  fpDataType=boolean  BlockIOType=Inport  DeviceType=0
  in_DigitalInputs.IN_DIG_28 : KIBES_Signal/KIBES_Signal  MBDS_LibraryBlock=on  DatabaseKey=459  SignalName=DigitalInputs.IN_DIG_28  SymbolName=DigitalInputs_IN_DIG_28_000459  DataType=boolean  Init=0  Slope=1  Bias=0  DataSize=1  fpDataType=boolean  BlockIOType=Inport  DeviceType=0
  in_DigitalInputs.IN_DIG_29 : KIBES_Signal/KIBES_Signal  MBDS_LibraryBlock=on  DatabaseKey=460  SignalName=DigitalInputs.IN_DIG_29  SymbolName=DigitalInputs_IN_DIG_29_000460  DataType=boolean  Init=0  Slope=1  Bias=0  DataSize=1  fpDataType=boolean  BlockIOType=Inport  DeviceType=0
  in_DigitalInputs.IN_DIG_30 : KIBES_Signal/KIBES_Signal  MBDS_LibraryBlock=on  DatabaseKey=480  SignalName=DigitalInputs.IN_DIG_30  SymbolName=DigitalInputs_IN_DIG_30_000480  DataType=boolean  Init=0  Slope=1  Bias=0  DataSize=1  fpDataType=boolean  BlockIOType=Inport  DeviceType=0
  in_DigitalInputs.IN_DIG_31 : KIBES_Signal/KIBES_Signal  MBDS_LibraryBlock=on  DatabaseKey=481  SignalName=DigitalInputs.IN_DIG_31  SymbolName=DigitalInputs_IN_DIG_31_000481  DataType=boolean  Init=0  Slope=1  Bias=0  DataSize=1  fpDataType=boolean  BlockIOType=Inport  DeviceType=0
  in_DigitalInputs.IN_DIG_32 : KIBES_Signal/KIBES_Signal  MBDS_LibraryBlock=on  DatabaseKey=482  SignalName=DigitalInputs.IN_DIG_32  SymbolName=DigitalInputs_IN_DIG_32_000482  DataType=boolean  Init=0  Slope=1  Bias=0  DataSize=1  fpDataType=boolean  BlockIOType=Inport  DeviceType=0
  in_DigitalInputs.IN_DIG_33 : KIBES_Signal/KIBES_Signal  MBDS_LibraryBlock=on  DatabaseKey=483  SignalName=DigitalInputs.IN_DIG_33  SymbolName=DigitalInputs_IN_DIG_33_000483  DataType=boolean  Init=0  Slope=1  Bias=0  DataSize=1  fpDataType=boolean  BlockIOType=Inport  DeviceType=0
  in_DigitalInputs.IN_DIG_34 : KIBES_Signal/KIBES_Signal  MBDS_LibraryBlock=on  DatabaseKey=484  SignalName=DigitalInputs.IN_DIG_34  SymbolName=DigitalInputs_IN_DIG_34_000484  DataType=boolean  Init=0  Slope=1  Bias=0  DataSize=1  fpDataType=boolean  BlockIOType=Inport  DeviceType=0
  in_DigitalInputs.IN_DIG_37 : KIBES_Signal/KIBES_Signal  MBDS_LibraryBlock=on  DatabaseKey=485  SignalName=DigitalInputs.IN_DIG_37  SymbolName=DigitalInputs_IN_DIG_37_000485  DataType=boolean  Init=0  Slope=1  Bias=0  DataSize=1  fpDataType=boolean  BlockIOType=Inport  DeviceType=0
  in_DigitalInputs.IN_DIG_38 : KIBES_Signal/KIBES_Signal  MBDS_LibraryBlock=on  DatabaseKey=486  SignalName=DigitalInputs.IN_DIG_38  SymbolName=DigitalInputs_IN_DIG_38_000486  DataType=boolean  Init=0  Slope=1  Bias=0  DataSize=1  fpDataType=boolean  BlockIOType=Inport  DeviceType=0
  in_DigitalInputs.IN_DIG_39 : KIBES_Signal/KIBES_Signal  MBDS_LibraryBlock=on  DatabaseKey=487  SignalName=DigitalInputs.IN_DIG_39  SymbolName=DigitalInputs_IN_DIG_39_000487  DataType=boolean  Init=0  Slope=1  Bias=0  DataSize=1  fpDataType=boolean  BlockIOType=Inport  DeviceType=0
  in_DigitalInputs.IN_DIG_41 : KIBES_Signal/KIBES_Signal  MBDS_LibraryBlock=on  DatabaseKey=488  SignalName=DigitalInputs.IN_DIG_41  SymbolName=DigitalInputs_IN_DIG_41_000488  DataType=boolean  Init=0  Slope=1  Bias=0  DataSize=1  fpDataType=boolean  BlockIOType=Inport  DeviceType=0
  in_DigitalInputs.IN_DIG_42 : KIBES_Signal/KIBES_Signal  MBDS_LibraryBlock=on  DatabaseKey=489  SignalName=DigitalInputs.IN_DIG_42  SymbolName=DigitalInputs_IN_DIG_42_000489  DataType=boolean  Init=0  Slope=1  Bias=0  DataSize=1  fpDataType=boolean  BlockIOType=Inport  DeviceType=0
  in_DigitalInputs.IN_DIG_43 : KIBES_Signal/KIBES_Signal  MBDS_LibraryBlock=on  DatabaseKey=490  SignalName=DigitalInputs.IN_DIG_43  SymbolName=DigitalInputs_IN_DIG_43_000490  DataType=boolean  Init=0  Slope=1  Bias=0  DataSize=1  fpDataType=boolean  BlockIOType=Inport  DeviceType=0
  in_DigitalInputs.IN_DIG_44 : KIBES_Signal/KIBES_Signal  MBDS_LibraryBlock=on  DatabaseKey=491  SignalName=DigitalInputs.IN_DIG_44  SymbolName=DigitalInputs_IN_DIG_44_000491  DataType=boolean  Init=0  Slope=1  Bias=0  DataSize=1  fpDataType=boolean  BlockIOType=Inport  DeviceType=0
  in_DigitalInputs.IN_DIG_45 : KIBES_Signal/KIBES_Signal  MBDS_LibraryBlock=on  DatabaseKey=492  SignalName=DigitalInputs.IN_DIG_45  SymbolName=DigitalInputs_IN_DIG_45_000492  DataType=boolean  Init=0  Slope=1  Bias=0  DataSize=1  fpDataType=boolean  BlockIOType=Inport  DeviceType=0
  in_DigitalInputs.IN_DIG_46 : KIBES_Signal/KIBES_Signal  MBDS_LibraryBlock=on  DatabaseKey=493  SignalName=DigitalInputs.IN_DIG_46  SymbolName=DigitalInputs_IN_DIG_46_000493  DataType=boolean  Init=0  Slope=1  Bias=0  DataSize=1  fpDataType=boolean  BlockIOType=Inport  DeviceType=0
  in_DigitalInputs.IN_DIG_48 : KIBES_Signal/KIBES_Signal  MBDS_LibraryBlock=on  DatabaseKey=494  SignalName=DigitalInputs.IN_DIG_48  SymbolName=DigitalInputs_IN_DIG_48_000494  DataType=boolean  Init=0  Slope=1  Bias=0  DataSize=1  fpDataType=boolean  BlockIOType=Inport  DeviceType=0
  in_DigitalInputs.IN_DIG_49 : KIBES_Signal/KIBES_Signal  MBDS_LibraryBlock=on  DatabaseKey=495  SignalName=DigitalInputs.IN_DIG_49  SymbolName=DigitalInputs_IN_DIG_49_000495  DataType=boolean  Init=0  Slope=1  Bias=0  DataSize=1  fpDataType=boolean  BlockIOType=Inport  DeviceType=0
  in_DigitalInputs.IN_DIG_50 : KIBES_Signal/KIBES_Signal  MBDS_LibraryBlock=on  DatabaseKey=496  SignalName=DigitalInputs.IN_DIG_50  SymbolName=DigitalInputs_IN_DIG_50_000496  DataType=boolean  Init=0  Slope=1  Bias=0  DataSize=1  fpDataType=boolean  BlockIOType=Inport  DeviceType=0
  in_IN_DIG_02_DriverDoor : KIBES_Signal/KIBES_Signal  MBDS_LibraryBlock=on  DatabaseKey=215  SignalName=IN_DIG_02_DriverDoor  SymbolName=IN_DIG_02_DriverDoor_000215  DataType=boolean  Init=0  Slope=1  Bias=0  DataSize=1  fpDataType=boolean  BlockIOType=Inport  DeviceType=0
  in_IN_DIG_10_CabinLight : KIBES_Signal/KIBES_Signal  MBDS_LibraryBlock=on  DatabaseKey=213  SignalName=IN_DIG_10_CabinLight  SymbolName=IN_DIG_10_CabinLight_000213  DataType=boolean  Init=0  Slope=1  Bias=0  DataSize=1  fpDataType=boolean  BlockIOType=Inport  DeviceType=0
  in_IN_DIG_17_Cabin_Lock : KIBES_Signal/KIBES_Signal  MBDS_LibraryBlock=on  DatabaseKey=211  SignalName=IN_DIG_17_Cabin_Lock  SymbolName=IN_DIG_17_Cabin_Lock_000211  DataType=boolean  Init=0  Slope=1  Bias=0  DataSize=1  fpDataType=boolean  BlockIOType=Inport  DeviceType=0
  in_IN_DIG_26_HazardSwitch : KIBES_Signal/KIBES_Signal  MBDS_LibraryBlock=on  DatabaseKey=212  SignalName=IN_DIG_26_HazardSwitch  SymbolName=IN_DIG_26_HazardSwitch_000212  DataType=boolean  Init=0  Slope=1  Bias=0  DataSize=1  fpDataType=boolean  BlockIOType=Inport  DeviceType=0
  in_IN_DIG_35_PassengerDoor : KIBES_Signal/KIBES_Signal  MBDS_LibraryBlock=on  DatabaseKey=214  SignalName=IN_DIG_35_PassengerDoor  SymbolName=IN_DIG_35_PassengerDoor_000214  DataType=boolean  Init=0  Slope=1  Bias=0  DataSize=1  fpDataType=boolean  BlockIOType=Inport  DeviceType=0
  in_IN_DIG_36_KL15 : KIBES_Signal/KIBES_Signal  MBDS_LibraryBlock=on  DatabaseKey=216  SignalName=IN_DIG_36_KL15  SymbolName=IN_DIG_36_KL15_000216  DataType=boolean  Init=0  Slope=1  Bias=0  DataSize=1  fpDataType=boolean  BlockIOType=Inport  DeviceType=0
  in_IN_DIG_40_KL58 : KIBES_Signal/KIBES_Signal  MBDS_LibraryBlock=on  DatabaseKey=210  SignalName=IN_DIG_40_KL58  SymbolName=IN_DIG_40_KL58_000210  DataType=boolean  Init=0  Slope=1  Bias=0  DataSize=1  fpDataType=boolean  BlockIOType=Inport  DeviceType=0
  in_IN_DigitalInputs.IN_DIG_01 : KIBES_Signal/KIBES_Signal  MBDS_LibraryBlock=on  DatabaseKey=73  SignalName=IN_DigitalInputs.IN_DIG_01  SymbolName=IN_DigitalInputs_IN_DIG_01_000073  DataType=boolean  Init=0  Slope=1  Bias=0  DataSize=1  fpDataType=boolean  BlockIOType=Inport  DeviceType=0
